simulink model "CalebsModel_v5"  (Simulink 8.3)
settings: Solver=ode45  StartTime=0.0  StopTime=StopTime  MaxStep=MaxStepSize  MinStep=MinStepSize  RelTol=RelTol
values from neighbouring files (symbols this model uses):
  a_lim = 0.008    [ControlDesign.m]
  b_surf = 1e3    (= 1000)    [ControlDesign.m]
  ba = (-(z_1*z_2*z_3)*Mar_hat + Mar_hat)/Ts    [ControlDesign.m]
  bo = (-(z_1*z_2*z_3)*Mar_hat + Mar_hat)/Ts    [ControlDesign.m]
  bp = 1    [ControlDesign.m]
  ContactPoint = 0.023    [ControlDesign.m]
  F_act_cmd = 25    [ControlDesign.m]
  F_ramp_slope = 5    [ControlDesign.m]
  F_time = 5    [ControlDesign.m]
  k_1 = (z_1*z_2-1+k_2*Ts)/(k_2*Ts^2)    [ControlDesign.m]
  k_2 = (2-(z_1+z_2))/Ts    [ControlDesign.m]
  K_backemf = 1000*mean( K_backemf_array )    [ControlDesign.m]
  K_L12_Force = 0.00229181    [ControlDesign.m]    (also in ControlDesignForceModeLinear.m = 2.29181)
  K_PWM = PWM_res/V_rail    (= 83.3333333333)    [ControlDesign.m]    (also in ControlDesignForceModeLinear.m = 0.012)
  k_surf = 1e7    (= 10000000)    [ControlDesign.m]
  kisa = (-(z_1 + z_2 + z_3)*Mar_hat + 3*Mar_hat - Ts*ba - (Ts^2)*ksa)/(Ts^3)    [ControlDesign.m]
  kiso = (-(z_1 + z_2 + z_3)*Mar_hat + 3*Mar_hat - Ts*bo - (Ts^2)*kso)/(Ts^3)    [ControlDesign.m]
  ksa = (-(z_1*z_2 + z_1*z_3 + z_2*z_3)*Mar_hat + 3*Mar_hat - 2*Ts*ba)/(Ts^2)    [ControlDesign.m]
  kso = (-(z_1*z_2 + z_1*z_3 + z_2*z_3)*Mar_hat + 3*Mar_hat - 2*Ts*bo)/(Ts^2)    [ControlDesign.m]
  kvc = 0.1    [ControlDesign.m]
  L12_Offset_I = 0.012995    [ControlDesign.m]    (also in ControlDesignForceModeLinear.m = 12.995)
  Mar = 0.075    [ControlDesign.m]    (also in ControlDesignForceModeLinear.m)
  Mar_hat = Mar    (= 0.075)    [ControlDesign.m]
  PositionCmdErr = -0.001    [ControlDesign.m]
  PWM_res = 2000    [ControlDesign.m]    (also in ControlDesignForceModeLinear.m)
  Ra_L12 = 60    [ControlDesign.m]    (also in ControlDesignForceModeLinear.m)
  Ts = 1/fs    (= 0.001)    [ControlDesign.m]    (also in ControlDesignForceModeLinear.m)
  v_lim = 0.003    [ControlDesign.m]
  ymod = 0.75e-3    (= 0.00075)    [ControlDesign.m]
undefined symbols (not defined in the file or in its folder): DiscIntNeverNeededParam
libraries: simulink x5
settings Model: Creator=secrest  LastModifiedBy=oberstare
settings SolverCC: AlgebraicLoopSolver=LineSearch
settings DataIOCC: SignalLoggingSaveFormat=Dataset
settings DebuggingCC: UnderspecifiedInitializationDetection=Simplified  FcnCallInpInsideContextMsg=UseLocalSettings  StateNameClashWarn=none

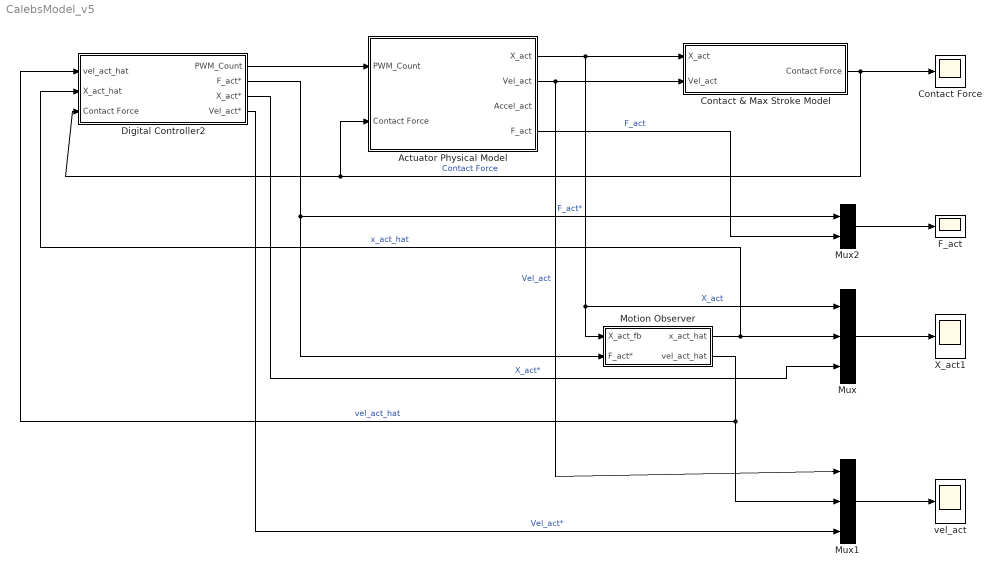
== system CalebsModel_v5 ==
  Actuator Physical Model : Subsystem
  Contact & Max Stroke Model : Subsystem
  Contact Force : Scope
      settings: ShowLegends=on  YMin=0  YMax=27.5  Decimation=100
  Digital Controller2 : Subsystem
  F_act : Scope
      settings: ShowLegends=on  YMin=-30  YMax=65  SaveName=ScopeData5
  Motion Observer : Subsystem
  Mux : Mux  Inputs=3
  Mux1 : Mux  Inputs=3
  Mux2 : Mux  Inputs=2
  X_act1 : Scope
      settings: ShowLegends=on  YMin=0  YMax=0.00325  SaveName=ScopeData2
  vel_act : Scope
      settings: ShowLegends=on  YMin=-0.0175  YMax=0.015  SaveName=ScopeData3
  wires:
  Digital Controller2/1(PWM_Count) -> Actuator Physical Model/1(PWM_Count)
  Actuator Physical Model/1(X_act) -> Motion Observer/1(X_act_fb), Mux/1, Contact & Max Stroke Model/1(X_act)  "X_act"
  Actuator Physical Model/2(Vel_act) -> Mux1/1, Contact & Max Stroke Model/2(Vel_act)  "Vel_act"
  Contact & Max Stroke Model/1(Contact Force) -> Contact Force/1, Actuator Physical Model/2(Contact Force), Digital Controller2/3(Contact Force)  "Contact Force"
  Motion Observer/1(x_act_hat) -> Mux/2, Digital Controller2/2(X_act_hat)  "x_act_hat"
  Mux/1 -> X_act1/1
  Mux1/1 -> vel_act/1
  Motion Observer/2(vel_act_hat) -> Mux1/2, Digital Controller2/1(vel_act_hat)  "vel_act_hat"
  Digital Controller2/2(F_act*) -> Motion Observer/2(F_act*), Mux2/1  "F_act*"
  Digital Controller2/3(X_act*) -> Mux/3  "X_act*"
  Mux2/1 -> F_act/1
  Actuator Physical Model/4(F_act) -> Mux2/2  "F_act"
  Digital Controller2/4(Vel_act*) -> Mux1/3  "Vel_act*"

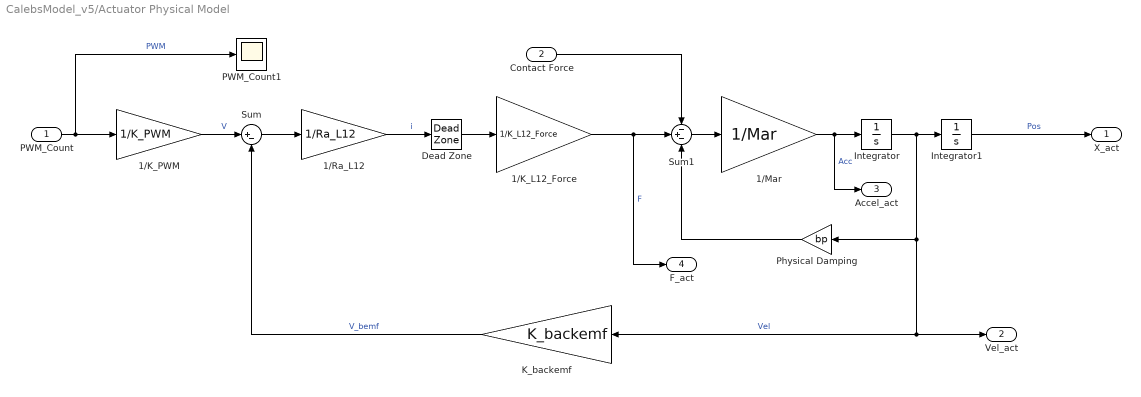
== system CalebsModel_v5/Actuator Physical Model ==
  PWM_Count : Inport
  Contact Force : Inport  Port=2
  1/K_L12_Force : Gain  Gain=1/K_L12_Force
  1/K_PWM : Gain  Gain=1/K_PWM
  1/Mar : Gain  Gain=1/Mar
  1/Ra_L12 : Gain  Gain=1/Ra_L12
  Dead Zone : DeadZone  LowerValue=-L12_Offset_I  UpperValue=L12_Offset_I  SaturateOnIntegerOverflow=on
  Integrator : Integrator
  Integrator1 : Integrator
  K_backemf : Gain  Gain=K_backemf
  PWM_Count1 : Scope
      settings: ShowLegends=on  YMin=-75  YMax=450  SaveName=ScopeData7
  Physical Damping : Gain  Gain=bp
  Sum : Sum  Inputs=|+-
  Sum1 : Sum  Inputs=-+-
  X_act : Outport
  Vel_act : Outport  Port=2
  Accel_act : Outport  Port=3
  F_act : Outport  Port=4
  wires:
  Sum1/1 -> 1/Mar/1
  1/Ra_L12/1 -> Dead Zone/1  "i"
  1/K_PWM/1 -> Sum/1  "V"
  Sum/1 -> 1/Ra_L12/1
  1/K_L12_Force/1 -> Sum1/2, F_act/1  "F"
  Integrator1/1 -> X_act/1  "Pos"
  Integrator/1 -> Integrator1/1, Physical Damping/1, K_backemf/1, Vel_act/1  "Vel"
  Contact Force/1 -> Sum1/1
  1/Mar/1 -> Accel_act/1, Integrator/1  "Acc"
  PWM_Count/1 -> PWM_Count1/1, 1/K_PWM/1  "PWM"
  Dead Zone/1 -> 1/K_L12_Force/1
  Physical Damping/1 -> Sum1/3
  K_backemf/1 -> Sum/2  "V_bemf"

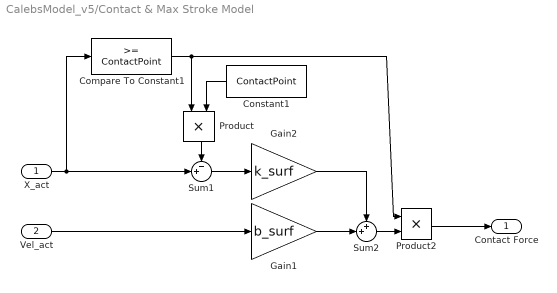
== system CalebsModel_v5/Contact & Max Stroke Model ==
  X_act : Inport
  Vel_act : Inport  Port=2
  Compare To Constant1 : simulink/Logic and Bit Operations/Compare To Constant  relop=>=  const=ContactPoint  OutDataTypeStr=uint8
  Constant1 : Constant  Value=ContactPoint
  Gain1 : Gain  Gain=b_surf
  Gain2 : Gain  Gain=k_surf
  Product : Product  RndMeth=Zero
  Product2 : Product  RndMeth=Zero
  Sum1 : Sum  Inputs=-+|
  Sum2 : Sum  Inputs=++|
  Contact Force : Outport
  wires:
  X_act/1 -> Sum1/2, Compare To Constant1/1
  Vel_act/1 -> Gain1/1
  Sum1/1 -> Gain2/1
  Constant1/1 -> Product/2
  Gain2/1 -> Sum2/1
  Gain1/1 -> Sum2/2
  Sum2/1 -> Product2/2
  Product2/1 -> Contact Force/1
  Compare To Constant1/1 -> Product/1, Product2/1
  Product/1 -> Sum1/1

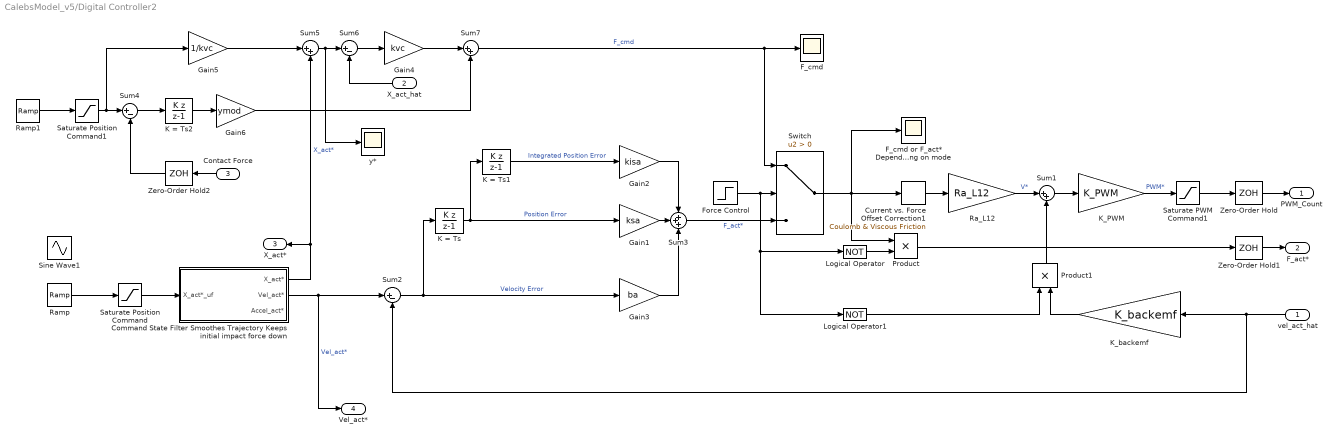
== system CalebsModel_v5/Digital Controller2 ==
  vel_act_hat : Inport
  X_act_hat : Inport  Port=2
  Contact Force : Inport  Port=3
  Command State Filter Smoothes Trajectory Keeps initial impact force down : Subsystem
  Current vs. Force Offset Correction1 : simulink/Discontinuities/Coulomb & Viscous Friction  offset=L12_Offset_I  gain=K_L12_Force
  F_cmd : Scope
      settings: YMax=5.5  SaveName=ScopeData4
  F_cmd or F_act* Depending on mode : Scope
      settings: YMax=5.5  SaveName=ScopeData9
  Force Control : Step  Time=F_time  SampleTime=0
  Gain1 : Gain  Gain=ksa
  Gain2 : Gain  Gain=kisa
  Gain3 : Gain  Gain=ba
  Gain4 : Gain  Gain=kvc
  Gain5 : Gain  Gain=1/kvc
  Gain6 : Gain  Gain=ymod
  K = Ts : DiscreteIntegrator  IntegratorMethod=Accumulation: Backward Euler  gainval=Ts  SampleTime=-1  ICPrevOutput=DiscIntNeverNeededParam  ICPrevScaledInput=DiscIntNeverNeededParam
  K = Ts1 : DiscreteIntegrator  IntegratorMethod=Accumulation: Backward Euler  gainval=Ts  SampleTime=-1  ICPrevOutput=DiscIntNeverNeededParam  ICPrevScaledInput=DiscIntNeverNeededParam
  K = Ts2 : DiscreteIntegrator  IntegratorMethod=Accumulation: Backward Euler  gainval=Ts  SampleTime=-1  ICPrevOutput=DiscIntNeverNeededParam  ICPrevScaledInput=DiscIntNeverNeededParam
  K_PWM : Gain  Gain=K_PWM
  K_backemf : Gain  Gain=K_backemf
  Logical Operator : Logic  Operator=NOT  AllPortsSameDT=off  OutDataTypeStr=boolean
  Logical Operator1 : Logic  Operator=NOT  AllPortsSameDT=off  OutDataTypeStr=boolean
  Product : Product  RndMeth=Zero
  Product1 : Product  RndMeth=Zero
  Ra_L12 : Gain  Gain=Ra_L12
  Ramp : simulink/Sources/Ramp  slope=0.8*v_lim  start=1  X0=0
  Ramp1 : simulink/Sources/Ramp  slope=F_ramp_slope  start=F_time  X0=0
  Saturate Position Command : Saturate  UpperLimit=ContactPoint+PositionCmdErr  LowerLimit=0  SampleTime=Ts
  Saturate Position Command1 : Saturate  UpperLimit=F_act_cmd  LowerLimit=0  SampleTime=Ts
  Saturate PWM Command1 : Saturate  UpperLimit=PWM_res  LowerLimit=-PWM_res
  Sine Wave1 : Sin  Amplitude=0.0001  Frequency=2*pi*1  SampleTime=Ts
  Sum1 : Sum  Inputs=|++
  Sum2 : Sum  Inputs=|+-
  Sum3 : Sum  Inputs=+++
  Sum4 : Sum  Inputs=|+-
  Sum5 : Sum  Inputs=|++
  Sum6 : Sum  Inputs=|+-
  Sum7 : Sum  Inputs=|++
  Switch : Switch  Criteria=u2 > Threshold
  Zero-Order Hold : ZeroOrderHold  SampleTime=Ts
  Zero-Order Hold1 : ZeroOrderHold  SampleTime=Ts
  Zero-Order Hold2 : ZeroOrderHold  SampleTime=Ts
  y* : Scope
      settings: YMin=0  YMax=17  SaveName=ScopeData8
  PWM_Count : Outport
  F_act* : Outport  Port=2
  X_act* : Outport  Port=3
  Vel_act* : Outport  Port=4
  wires:
  K_PWM/1 -> Saturate PWM Command1/1  "PWM*"
  Ra_L12/1 -> Sum1/1  "V*"
  Sum1/1 -> K_PWM/1
  vel_act_hat/1 -> K_backemf/1, Sum2/2
  Zero-Order Hold/1 -> PWM_Count/1
  Zero-Order Hold1/1 -> F_act*/1
  Current vs. Force Offset Correction1/1 -> Ra_L12/1
  Sum2/1 -> Gain3/1, K = Ts/1  "Velocity Error"
  Gain2/1 -> Sum3/1
  Gain1/1 -> Sum3/2
  Gain3/1 -> Sum3/3
  K = Ts/1 -> Gain1/1, K = Ts1/1  "Position Error"
  K = Ts1/1 -> Gain2/1  "Integrated Position Error"
  Command State Filter Smoothes Trajectory Keeps initial impact force down/2(Vel_act*) -> Sum2/1, Vel_act*/1  "Vel_act*"
  Command State Filter Smoothes Trajectory Keeps initial impact force down/1(X_act*) -> X_act*/1, Sum5/2  "X_act*"
  Saturate PWM Command1/1 -> Zero-Order Hold/1
  Ramp/1 -> Saturate Position Command/1
  Saturate Position Command/1 -> Command State Filter Smoothes Trajectory Keeps initial impact force down/1(X_act*_uf)
  Switch/1 -> Current vs. Force Offset Correction1/1, Product/1, F_cmd or F_act* Depending on mode/1
  Sum3/1 -> Switch/3  "F_act*"
  Contact Force/1 -> Zero-Order Hold2/1
  Gain5/1 -> Sum5/1
  Sum4/1 -> K = Ts2/1
  Sum5/1 -> Sum6/1, y*/1
  Sum6/1 -> Gain4/1
  Gain4/1 -> Sum7/1
  K = Ts2/1 -> Gain6/1
  Gain6/1 -> Sum7/2
  Sum7/1 -> Switch/1, F_cmd/1  "F_cmd"
  Force Control/1 -> Switch/2, Logical Operator/1, Logical Operator1/1
  Zero-Order Hold2/1 -> Sum4/2
  Product/1 -> Zero-Order Hold1/1
  Logical Operator/1 -> Product/2
  X_act_hat/1 -> Sum6/2
  Ramp1/1 -> Saturate Position Command1/1
  Saturate Position Command1/1 -> Sum4/1, Gain5/1
  Product1/1 -> Sum1/2
  K_backemf/1 -> Product1/2
  Logical Operator1/1 -> Product1/1

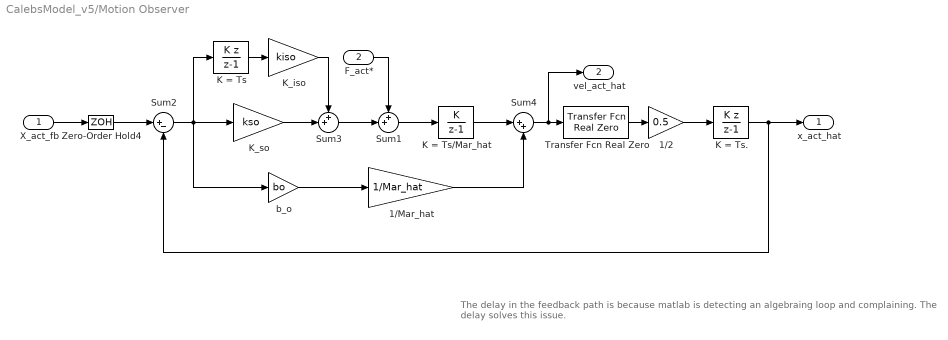
== system CalebsModel_v5/Motion Observer ==
  note: The delay in the feedback path is because matlab is detecting an algebraing loop and complaining.
      | The delay solves this issue.
  X_act_fb : Inport
  F_act* : Inport  Port=2
  1/2 : Gain  Gain=0.5
  1/Mar_hat : Gain  Gain=1/Mar_hat
  K = Ts : DiscreteIntegrator  IntegratorMethod=Accumulation: Backward Euler  gainval=Ts  SampleTime=-1  ICPrevOutput=DiscIntNeverNeededParam  ICPrevScaledInput=DiscIntNeverNeededParam
  K = Ts. : DiscreteIntegrator  IntegratorMethod=Accumulation: Backward Euler  gainval=Ts  SampleTime=-1  ICPrevOutput=DiscIntNeverNeededParam  ICPrevScaledInput=DiscIntNeverNeededParam
  K = Ts/Mar_hat : DiscreteIntegrator  IntegratorMethod=Accumulation: Forward Euler  gainval=Ts/Mar_hat  SampleTime=-1  ICPrevOutput=DiscIntNeverNeededParam  ICPrevScaledInput=DiscIntNeverNeededParam
  K_iso : Gain  Gain=kiso
  K_so : Gain  Gain=kso
  Sum1 : Sum  Inputs=++|
  Sum2 : Sum  Inputs=|+-
  Sum3 : Sum  Inputs=++|
  Sum4 : Sum  Inputs=|++
  Transfer Fcn Real Zero : simulink/Discrete/Transfer Fcn Real Zero  ZeroZ=-1  ICPrevInput=0.0  InputProcessing=Inherited  DoSatur=off
  Zero-Order Hold4 : ZeroOrderHold  SampleTime=Ts
  b_o : Gain  Gain=bo
  x_act_hat : Outport
  vel_act_hat : Outport  Port=2
  wires:
  K = Ts/1 -> K_iso/1
  K_iso/1 -> Sum3/1
  b_o/1 -> 1/Mar_hat/1
  Sum1/1 -> K = Ts/Mar_hat/1
  K = Ts/Mar_hat/1 -> Sum4/1
  Sum4/1 -> Transfer Fcn Real Zero/1, vel_act_hat/1
  Transfer Fcn Real Zero/1 -> 1/2/1
  1/2/1 -> K = Ts./1
  K = Ts./1 -> x_act_hat/1, Sum2/2
  X_act_fb/1 -> Zero-Order Hold4/1
  K_so/1 -> Sum3/2
  Sum2/1 -> K_so/1, K = Ts/1, b_o/1
  Zero-Order Hold4/1 -> Sum2/1
  Sum3/1 -> Sum1/2
  1/Mar_hat/1 -> Sum4/2
  F_act*/1 -> Sum1/1

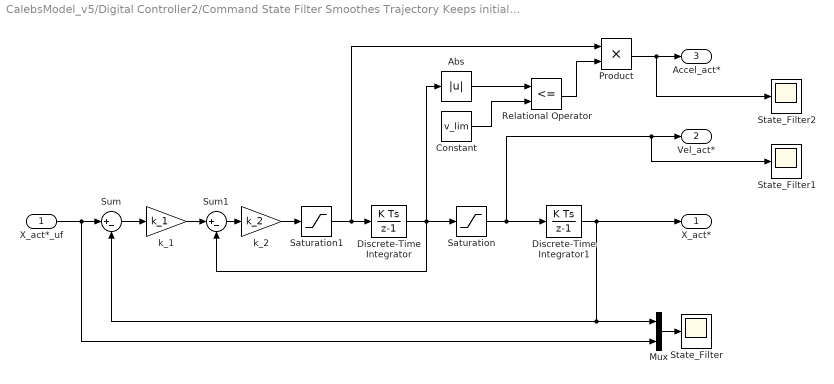
== system CalebsModel_v5/Digital Controller2/Command State Filter Smoothes Trajectory Keeps initial impact force down ==
  X_act*_uf : Inport
  Abs : Abs
  Constant : Constant  Value=v_lim
  Discrete-Time Integrator : DiscreteIntegrator  SampleTime=-1  ICPrevOutput=DiscIntNeverNeededParam  ICPrevScaledInput=DiscIntNeverNeededParam
  Discrete-Time Integrator1 : DiscreteIntegrator  SampleTime=-1  ICPrevOutput=DiscIntNeverNeededParam  ICPrevScaledInput=DiscIntNeverNeededParam
  Mux : Mux  Inputs=2
  Product : Product  RndMeth=Zero
  Relational Operator : RelationalOperator  Operator=<=  OutDataTypeStr=boolean
  Saturation : Saturate  UpperLimit=v_lim  LowerLimit=-v_lim
  Saturation1 : Saturate  UpperLimit=a_lim  LowerLimit=-a_lim
  State_Filter : Scope
      settings: YMin=0  YMax=0.002  SaveName=ScopeData2
  State_Filter1 : Scope
      settings: YMin=-0.0001  YMax=0.0001
  State_Filter2 : Scope
      settings: YMin=-0.006  YMax=0.006  SaveName=ScopeData6
  Sum : Sum  Inputs=|+-
  Sum1 : Sum  Inputs=|+-
  k_1 : Gain  Gain=k_1
  k_2 : Gain  Gain=k_2
  X_act* : Outport
  Vel_act* : Outport  Port=2
  Accel_act* : Outport  Port=3
  wires:
  Sum/1 -> k_1/1
  k_1/1 -> Sum1/1
  Sum1/1 -> k_2/1
  k_2/1 -> Saturation1/1
  Discrete-Time Integrator/1 -> Sum1/2, Saturation/1, Abs/1
  Discrete-Time Integrator1/1 -> X_act*/1, Sum/2, Mux/1
  Abs/1 -> Relational Operator/1
  Constant/1 -> Relational Operator/2
  Product/1 -> Accel_act*/1, State_Filter2/1
  Saturation/1 -> Discrete-Time Integrator1/1, Vel_act*/1, State_Filter1/1
  Saturation1/1 -> Discrete-Time Integrator/1, Product/1
  Mux/1 -> State_Filter/1
  X_act*_uf/1 -> Sum/1, Mux/2
  Relational Operator/1 -> Product/2
